simulink model "LR_2_var2"  (R2020b)
settings: Solver=FixedStepAuto  StartTime=0.0  StopTime=15  FixedStep=0.001  RelTol=1e-3
settings Model: Creator=SIA  LastModifiedBy=SIA

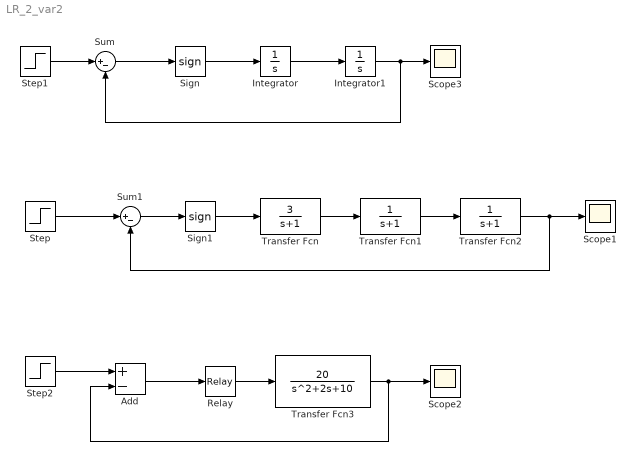
== system LR_2_var2 ==
  Add : Sum  Inputs=+-
  Integrator : Integrator
  Integrator1 : Integrator
  Relay : Relay  OnSwitchValue=0.5  OffSwitchValue=-0.5  OffOutputValue=-1
  Scope1 : Scope
  Scope2 : Scope
  Scope3 : Scope
  Sign : Signum
  Sign1 : Signum
  Step : Step  Time=0.01  Before=1  After=0  SampleTime=0
  Step1 : Step  Time=0.01  Before=1  After=0  SampleTime=0
  Step2 : Step  Time=0.01  Before=1  After=0  SampleTime=0
  Sum : Sum  Inputs=|+-
  Sum1 : Sum  Inputs=|+-
  Transfer Fcn : TransferFcn  Numerator=[3]  Denominator=[1 1]
  Transfer Fcn1 : TransferFcn  Denominator=[1 1]
  Transfer Fcn2 : TransferFcn  Denominator=[1 1]
  Transfer Fcn3 : TransferFcn  Numerator=[20]  Denominator=[1 2 10]
  wires:
  Sum/1 -> Sign/1
  Sign/1 -> Integrator/1
  Integrator/1 -> Integrator1/1
  Integrator1/1 -> Scope3/1, Sum/2
  Step1/1 -> Sum/1
  Sum1/1 -> Sign1/1
  Sign1/1 -> Transfer Fcn/1
  Transfer Fcn/1 -> Transfer Fcn1/1
  Transfer Fcn1/1 -> Transfer Fcn2/1
  Transfer Fcn2/1 -> Scope1/1, Sum1/2
  Step2/1 -> Add/1
  Add/1 -> Relay/1
  Relay/1 -> Transfer Fcn3/1
  Transfer Fcn3/1 -> Scope2/1, Add/2
  Step/1 -> Sum1/1
